simulink model "termproject_noideal"  (R2020a)
settings: Solver=VariableStepAuto  StartTime=0.0  StopTime=10.0  RelTol=1e-3
undefined symbols (not defined in the file): Acid, Lead
libraries: powerlib x28, electricdrivelib x1, simulink x1, eePwmGenerator x1, powerlib_meascontrol x1
settings Model: Creator=görkem  LastModifiedBy=görkem

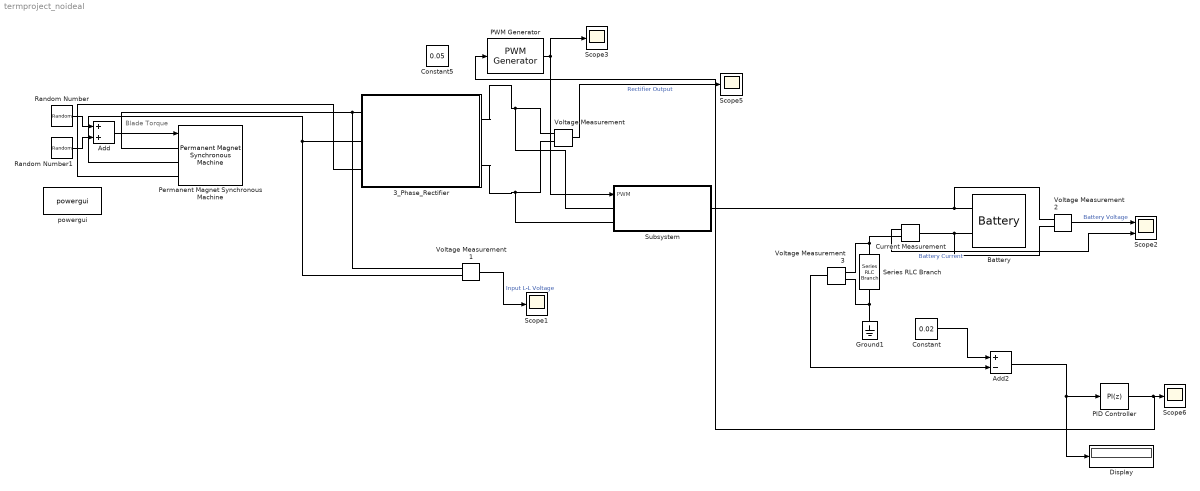
== system termproject_noideal ==
  note: Blade Torque
  3_Phase_Rectifier : Subsystem
  Add : Sum
  Add2 : Sum  Inputs=+-
  Battery : electricdrivelib/Extra Sources/Battery  BatType=Lead-Acid  ShowTempParam=off  ThermalPreset=no  ShowAgeParam=off  NomV=24  NomQ=5.4  SOC=50  Batt_Tr=30  PresetModel=on  MaxQ=5.625  MinV=18  FullV=26.1316  Dis_rate=1.08  R=0.044444  Normal_OP=1.6755  expZone="[24.4342        0.018]"  current=[6.5 13 32.5]  Units=Time  Tci=20  NomT=20  T2=-30  MaxQ2=4.8  FullV2=7.1  Normal_OP2=5.655  expZone2="[6.58           1]"  Rca=0.6  ti=2000  Dp=0  Neq0=0  Tsim=1e6  Ta1=25  Qeol=5.4*0.9  Reol=0.013333*1.2  Char_age=[2.3478, 3]  Dis_age=[2.3478, 10]  N1=1500  N2=10500  N3=1000  N4=1400  Ta2=45  N5=950
  Constant : Constant  Value=0.02
  Constant5 : Constant  Value=0.05
  Current Measurement : powerlib/Measurements/Current Measurement  PhasorSimulation=off  OutputType=Complex  PSBequivalent=0
  Display : Display
  Ground1 : powerlib/Elements/Ground  LConnTagsString=a
  PID Controller : simulink/Continuous/PID Controller  Controller=PI  Form=Parallel  TimeDomain=Discrete-time  UseExternalTs=off  SampleTime=0.0001  IntegratorMethod=Forward Euler  FilterMethod=Forward Euler  ControllerParametersSource=internal  P=45  I=10  D=0  UseFilter=on  N=100  TunerSelectOption=Transfer Function Based (PID Tuner App)  InitialConditionSource=internal  InitialConditionForIntegrator=0  InitialConditionForFilter=0  DifferentiatorICPrevScaledInput=0  ExternalReset=none  TrackingMode=off  Kt=1  LimitOutput=off  UpperSaturationLimit=inf  LowerSaturationLimit=-inf  LinearizeAsGain=on  AntiWindupMode=none  Kb=1  POutMin=[]  POutMax=[]  IOutMin=[]  IOutMax=[]  DOutMin=[]  DOutMax=[]  NOutMin=[]  NOutMax=[]  SumOutMin=[]  SumOutMax=[]  SaturationOutMin=[]  SaturationOutMax=[]  PParamMin=[]  PParamMax=[]  IParamMin=[]  IParamMax=[]  DParamMin=[]  DParamMax=[]  NParamMin=[]  NParamMax=[]  KbParamMin=[]  KbParamMax=[]  KtParamMin=[]  KtParamMax=[]  KbOutMin=[]  KbOutMax=[]  KtOutMin=[]  KtOutMax=[]  IntegratorOutMin=[]  IntegratorOutMax=[]  FilterOutMin=[]  FilterOutMax=[]  SumI1OutMin=[]  SumI1OutMax=[]  SumI2OutMin=[]  SumI2OutMax=[]  SumI3OutMin=[]  SumI3OutMax=[]  SumI4OutMin=[]  SumI4OutMax=[]  SumDOutMin=[]  SumDOutMax=[]  DifferentiatorOutMin=[]  DifferentiatorOutMax=[]  FilterDiffOutCoefMin=[]  FilterDiffOutCoefMax=[]  ReciprocalOutMin=[]  ReciprocalOutMax=[]  SumDenOutMin=[]  SumDenOutMax=[]  SumNumOutMin=[]  SumNumOutMax=[]  DivideOutMin=[]  DivideOutMax=[]  UdiffTsProdOutMin=[]  UdiffTsProdOutMax=[]  NTsProdOutMin=[]  NTsProdOutMax=[]  UintegralTsProdOutMin=[]  UintegralTsProdOutMax=[]  UngainTsProdOutMin=[]  UngainTsProdOutMax=[]  IntegratorContinuousStateAttributes=''  IntegratorStateMustResolveToSignalObject=off  IntegratorRTWStateStorageClass=Auto  FilterContinuousStateAttributes=''  FilterStateMustResolveToSignalObject=off  FilterRTWStateStorageClass=Auto  ParallelPVariant=InternalParameters  IdealPVariant=Disabled  IVariant=InternalParameters  DVariant=Disabled  IntegratorVariant=Discrete  SatVariant=Disabled  AWVariant=Passthrough  PCopyVariant=Disabled  TRVariant=Disabled  FdbkBlocksVariant=Forward  IdealPFdbkVariant=Disabled  SatFdbkVariant=Disabled  DerivativeFilterVariant=Disabled  NVariant=Disabled  NCopyVariant=Disabled_SignalSpec  FilterICVariant=Disabled  IntegratorICVariant=InternalICs  ExternalResetVariant=Disabled  TRSumVariant=Passthrough  SumFdbkVariant=Disabled  SumVariant=Sum_PI  TsampFilterVariant=InternalTs  TsampNgainVariant=Passthrough  TsampIntegralVariant=Passthrough
  PWM Generator : eePwmGenerator/PWM Generator  CarrCount=Up  Tper=0.0001  Ts=1e-5
  Permanent Magnet Synchronous Machine : powerlib/Machines/Permanent Magnet Synchronous Machine  NbPhases=3  FluxDistribution=Sinusoidal  RotorType=Round  MechanicalLoad=Torque Tm  PresetModel=No  ShowDetailedParameters=on  MeasurementBus=off  Resistance=10.58  Inductance=8.5e-3  dqInductances=[8.5e-3,8.5e-3]  La=0.0167  MachineConstant=Voltage Constant (V_peak L-L / krpm)  Flux=0.60646  VoltageCst=110  TorqueCst=0.90969  Flat=120  Mechanical=[0.00027 0.005024 1 0]  PolePairs=4  InitialConditions=[300,0, 0,0]  InitialConditions5ph=[0 0 0 0 0 0]  RefAngle=90 degrees behind phase A axis (modified Park)  IterativeDiscreteModel=Trapezoidal non iterative  TsBlock=-1  TsPowergui=0
  Random Number : RandomNumber  Mean=-1.6  Variance=0.05  SampleTime=1
  Random Number1 : RandomNumber  Variance=0.1  SampleTime=1e-3
  Scope{1,3,5..6} (4 alike) : Scope
  Scope2 : Scope  NumInputPorts=2
  Series RLC Branch : powerlib/Elements/Series RLC Branch  LConnTagsString=__new0  RConnTagsString=__new0  BranchType=R  Resistance=0.01  Inductance=1e-3  SetiL0=off  InitialCurrent=0  Capacitance=1e-6  Setx0=off  InitialVoltage=0  Measurements=None
  Subsystem : Subsystem
  Voltage Measurement{,1..3} (4 alike) : powerlib/Measurements/Voltage Measurement  PhasorSimulation=off  OutputType=Complex  PSBequivalent=0
  powergui : powerlib/powergui  Priority=1  SimulationMode=Discrete  SampleTime=1e-5  frequency=60  Iterations=50  frequencyindice=0  Pbase=100e6  ErrMax=1e-4  UnitsV=kV  UnitsW=MW  buscounter=0  FunctionMessages=off  echomessages=off  EnableUseOfTLC=off  CurrentSourceSwitches=off  DisableSnubberDevices=off  DisableRonSwitches=off  DisableVfSwitches=off  DisplayEquations=off  AutomaticDiscreteSolvers=off  SolverType=Tustin/Backward Euler (TBE)  Interpol=off  ExternalGateDelay=off  methode=off  Ts=100  x0status=blocks  SPID=on  SwTol=0  HookPort=off  NonlinearTolerance=1e-4  nMaxIteration=100  ContinueOnMaxIteration=off  RestoreLinks=warning  ResistiveCurrentMeasurement=off  Frange=[0:2:500]  Ylog=off  Xlog=on  ShowGrid=off  save=off  variable=ZData  structure=outputcurrent_rec  ZoomFFT=off  StartTime=0.0  cycles=1  DisplayStyle=1  fundamental=50  FreqAxis=off  MaxFrequency=1000  frequencyindicesteady=1  RmsSteady=1  display=off
  wires:
  Random Number/1 -> Add/1
  Voltage Measurement3/1 -> Add2/2
  Add2/1 -> Display/1, PID Controller/1
  Voltage Measurement2/1 -> Scope2/1  "Battery Voltage"
  Voltage Measurement/1 -> Scope5/1  "Rectifier Output"
  Random Number1/1 -> Add/2
  PWM Generator/1 -> Scope3/1, Subsystem/1(PWM)
  Add/1 -> Permanent Magnet Synchronous Machine/1
  Constant/1 -> Add2/1
  Voltage Measurement1/1 -> Scope1/1  "Input L-L Voltage"
  Current Measurement/1 -> Scope2/2  "Battery Current"
  PID Controller/1 -> PWM Generator/1, Scope6/1
  connections:
  Current Measurement/LConn1 -- Voltage Measurement2/LConn2 -- Battery/LConn2
  Ground1/LConn1 -- Series RLC Branch/RConn1 -- Voltage Measurement3/LConn2
  3_Phase_Rectifier/LConn2 -- Permanent Magnet Synchronous Machine/LConn2 -- Voltage Measurement1/LConn2
  Current Measurement/RConn1 -- Series RLC Branch/LConn1 -- Voltage Measurement3/LConn1
  Battery/LConn1 -- Voltage Measurement2/LConn1 -- Subsystem/RConn1
  Voltage Measurement/LConn1 -- 3_Phase_Rectifier/RConn1 -- Subsystem/LConn1
  3_Phase_Rectifier/LConn1 -- Permanent Magnet Synchronous Machine/LConn1 -- Voltage Measurement1/LConn1
  3_Phase_Rectifier/RConn2 -- Voltage Measurement/LConn2 -- Subsystem/LConn2
  Permanent Magnet Synchronous Machine/LConn3 -- 3_Phase_Rectifier/LConn3

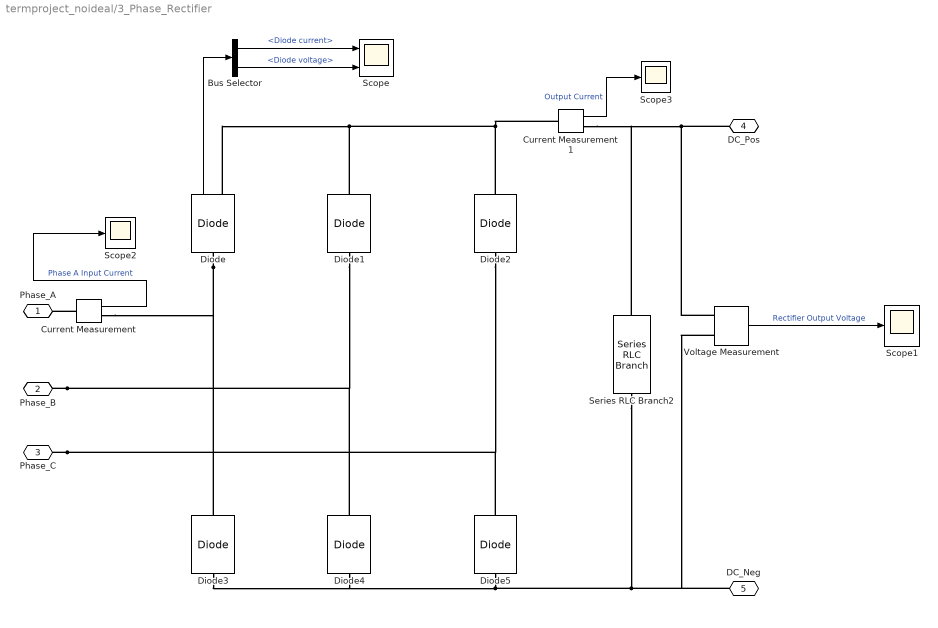
== system termproject_noideal/3_Phase_Rectifier ==
  Bus Selector : BusSelector  OutputSignals=Diode current,Diode voltage
  Current Measurement : powerlib/Measurements/Current Measurement  PhasorSimulation=off  OutputType=Complex  PSBequivalent=0
  Current Measurement1 : powerlib/Measurements/Current Measurement  PhasorSimulation=off  OutputType=Complex  PSBequivalent=0
  Diode : powerlib/Power Electronics/Diode  Ron=0.06  Lon=0  Vf=1.3  IC=0  UseSnubber=0  Rs=500  Cs=250e-9  Measurements=on
  Diode{1..5} (5 alike) : powerlib/Power Electronics/Diode  Ron=0.06  Lon=0  Vf=1.3  IC=0  UseSnubber=0  Rs=500  Cs=250e-9  Measurements=off
  Scope : Scope  NumInputPorts=2
  Scope1 : Scope
  Scope2 : Scope
  Scope3 : Scope
  Series RLC Branch2 : powerlib/Elements/Series RLC Branch  LConnTagsString=__new0  RConnTagsString=__new0  BranchType=C  Resistance=72  Inductance=1e-3  SetiL0=off  InitialCurrent=0  Capacitance=1e-3  Setx0=off  InitialVoltage=0  Measurements=None
  Voltage Measurement : powerlib/Measurements/Voltage Measurement  PhasorSimulation=off  OutputType=Complex  PSBequivalent=0
  Phase_A : PMIOPort  Side=Left
  Phase_B : PMIOPort  Port=2  Side=Left
  Phase_C : PMIOPort  Port=3  Side=Left
  DC_Pos : PMIOPort  Port=4  Side=Right
  DC_Neg : PMIOPort  Port=5  Side=Right
  wires:
  Diode/1 -> Bus Selector/1
  Bus Selector/1 -> Scope/1  "<Diode current>"
  Bus Selector/2 -> Scope/2  "<Diode voltage>"
  Voltage Measurement/1 -> Scope1/1  "Rectifier Output Voltage"
  Current Measurement1/1 -> Scope3/1  "Output Current"
  Current Measurement/1 -> Scope2/1  "Phase A Input Current"
  connections:
  Phase_C/RConn1 -- Diode5/RConn1 -- Diode2/LConn1
  Diode5/LConn1 -- Diode4/LConn1 -- Diode3/LConn1 -- Series RLC Branch2/RConn1 -- DC_Neg/RConn1 -- Voltage Measurement/LConn2
  Diode/LConn1 -- Diode3/RConn1 -- Current Measurement/RConn1
  Phase_B/RConn1 -- Diode4/RConn1 -- Diode1/LConn1
  Diode2/RConn1 -- Diode1/RConn1 -- Diode/RConn1 -- Current Measurement1/LConn1
  Current Measurement/LConn1 -- Phase_A/RConn1
  Voltage Measurement/LConn1 -- DC_Pos/RConn1 -- Series RLC Branch2/LConn1 -- Current Measurement1/RConn1

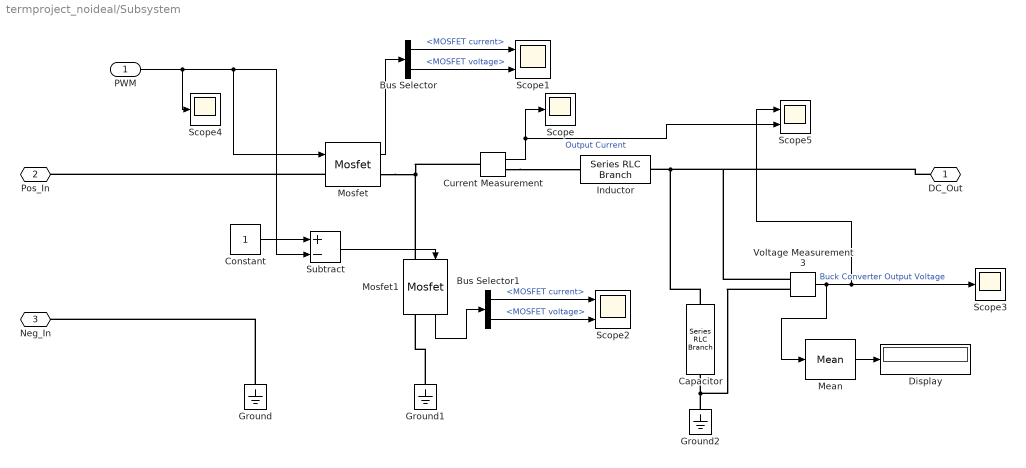
== system termproject_noideal/Subsystem ==
  PWM : Inport
  Bus Selector : BusSelector  OutputSignals=MOSFET current,MOSFET voltage
  Bus Selector1 : BusSelector  OutputSignals=MOSFET current,MOSFET voltage
  Capacitor : powerlib/Elements/Series RLC Branch  LConnTagsString=__new0  RConnTagsString=__new0  BranchType=C  Resistance=1  Inductance=1e-3  SetiL0=off  InitialCurrent=0  Capacitance=1e-3  Setx0=off  InitialVoltage=0  Measurements=None
  Constant : Constant
  Current Measurement : powerlib/Measurements/Current Measurement  PhasorSimulation=off  OutputType=Complex  PSBequivalent=0
  Display : Display
  Ground : powerlib/Elements/Ground  LConnTagsString=a
  Ground1 : powerlib/Elements/Ground  LConnTagsString=a
  Ground2 : powerlib/Elements/Ground  LConnTagsString=a
  Inductor : powerlib/Elements/Series RLC Branch  LConnTagsString=__new0  RConnTagsString=__new0  BranchType=L  Resistance=1  Inductance=5e-3  SetiL0=off  InitialCurrent=0  Capacitance=1e-6  Setx0=off  InitialVoltage=0  Measurements=None
  Mean : powerlib_meascontrol/Measurements/Mean  Freq=60  Vinit=0  Ts=0
  Mosfet : powerlib/Power Electronics/Mosfet  Ron=1.38  Lon=0  Rd=0.01  Vfd=1.4  IC=0  Rs=1e5  Cs=inf  Measurements=on
  Mosfet1 : powerlib/Power Electronics/Mosfet  Ron=1.38  Lon=0  Rd=0.01  Vfd=1.4  IC=0  Rs=1e5  Cs=inf  Measurements=on
  Scope : Scope
  Scope1 : Scope  NumInputPorts=2
  Scope2 : Scope  NumInputPorts=2
  Scope3 : Scope
  Scope4 : Scope
  Scope5 : Scope  NumInputPorts=2
  Subtract : Sum  Inputs=+-
  Voltage Measurement3 : powerlib/Measurements/Voltage Measurement  PhasorSimulation=off  OutputType=Complex  PSBequivalent=0
  DC_Out : PMIOPort  Side=Right
  Pos_In : PMIOPort  Port=2  Side=Left
  Neg_In : PMIOPort  Port=3  Side=Left
  wires:
  PWM/1 -> Subtract/2, Mosfet/1, Scope4/1
  Voltage Measurement3/1 -> Mean/1, Scope5/1, Scope3/1  "Buck Converter Output Voltage"
  Constant/1 -> Subtract/1
  Subtract/1 -> Mosfet1/1
  Current Measurement/1 -> Scope5/2, Scope/1  "Output Current"
  Mosfet/1 -> Bus Selector/1
  Bus Selector/1 -> Scope1/1  "<MOSFET current>"
  Bus Selector/2 -> Scope1/2  "<MOSFET voltage>"
  Mosfet1/1 -> Bus Selector1/1
  Bus Selector1/1 -> Scope2/1  "<MOSFET current>"
  Bus Selector1/2 -> Scope2/2  "<MOSFET voltage>"
  Mean/1 -> Display/1
  connections:
  Ground2/LConn1 -- Voltage Measurement3/LConn2 -- Capacitor/RConn1
  Current Measurement/LConn1 -- Mosfet/RConn1 -- Mosfet1/LConn1
  Capacitor/LConn1 -- Voltage Measurement3/LConn1 -- DC_Out/RConn1 -- Inductor/RConn1
  Ground1/LConn1 -- Mosfet1/RConn1
  Ground/LConn1 -- Neg_In/RConn1
  Current Measurement/RConn1 -- Inductor/LConn1
  Mosfet/LConn1 -- Pos_In/RConn1
